simulink model "Subsystem"  (R2018a)
settings: Solver=ode45  StartTime=0.0  StopTime=simTime  RelTol=1e-3
values from neighbouring files (symbols this model uses):
  Ki_m = 0.147819660015    [C_accel2.mat]    (also in simulation _old.m = double(sol.Kis(i)); simulation.m = double(sol.Kis(i)); simulation_moteur.m = double(sol.Kis(i)))
  Km = 1353    [C_accel.mat]    (also in C_accel2.mat; parametres.m = 1311.7; simulation _old.m = 1311.7; simulation.m = 1311.7)
  Kp_m = 0.0140428677014    [C_accel2.mat]    (also in simulation _old.m = double(sol.Kps(i)); simulation.m = double(sol.Kps(i)); simulation_moteur.m = double(sol.Kps(i)))
  Tau_m = 0.274    [C_accel.mat]    (also in C_accel2.mat; parametres.m = 0.205; simulation _old.m = 0.205; simulation.m = 0.205)
settings Model: Creator=chsira  LastModifiedBy=charl
settings SolverCC: MaxConsecutiveZCs=10000
settings DataIOCC: SaveOutput=off  SaveTime=off
settings DebuggingCC: MaxConsecutiveZCsMsg=none  LibraryContextMissingDiagnostic=warning
settings ModelReferenceCC: ModelReferenceMinAlgLoopOccurrences=on
settings SFSimCC: SimUseLocalCustomCode=on
settings RTWCC: RTWUseLocalCustomCode=on
settings GRTTargetCC: CombineOutputUpdateFcns=off

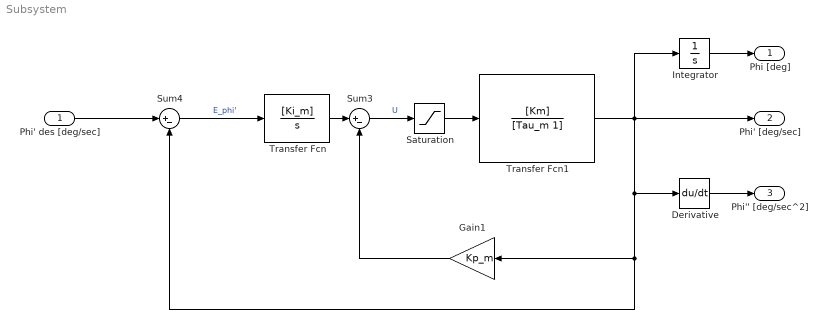
== system Subsystem ==
  Phi' des [deg/sec] : Inport  OutDataTypeStr=double  PortDimensions=1
  Derivative : Derivative
  Gain1 : Gain  Gain=Kp_m
  Integrator : Integrator
  Saturation : Saturate  UpperLimit=6  LowerLimit=-6
  Sum3 : Sum  Inputs=|+-
  Sum4 : Sum  Inputs=|+-
  Transfer Fcn : TransferFcn  Numerator=[Ki_m]  Denominator=[1 0]
  Transfer Fcn1 : TransferFcn  Numerator=[Km]  Denominator=[Tau_m 1]
  Phi [deg] : Outport  OutDataTypeStr=double  PortDimensions=1  SampleTime=0
  Phi' [deg/sec] : Outport  Port=2  OutDataTypeStr=double  PortDimensions=1  SampleTime=0
  Phi'' [deg/sec^2] : Outport  Port=3  OutDataTypeStr=double  PortDimensions=1  SampleTime=0
  wires:
  Phi' des [deg/sec]/1 -> Sum4/1
  Transfer Fcn1/1 -> Integrator/1, Derivative/1, Gain1/1, Sum4/2, Phi' [deg/sec]/1
  Sum4/1 -> Transfer Fcn/1  "E_phi'"
  Transfer Fcn/1 -> Sum3/1
  Sum3/1 -> Saturation/1  "U"
  Integrator/1 -> Phi [deg]/1
  Saturation/1 -> Transfer Fcn1/1
  Gain1/1 -> Sum3/2
  Derivative/1 -> Phi'' [deg/sec^2]/1
